simulink model "tetherDragForce_th"  (R2018b)
settings: Solver=VariableStepAuto  StartTime=0.0  StopTime=0  RelTol=1e-3
values from neighbouring files (symbols this model uses):
  flow = [1 0 0]'    [tetherDragForce_ts.m]
  R1_o = [0 0 0]'    [tetherDragForce_ts.m]
  Ri_o = zeros(3,N-2)    [tetherDragForce_ts.m]
  Rn_o = [0 0 100]'    [tetherDragForce_ts.m]
  V1_o = [0 0 0]'    [tetherDragForce_ts.m]
  Vi_o = zeros(size(Ri_o))    [tetherDragForce_ts.m]
  Vn_o = [0 0 0]'    [tetherDragForce_ts.m]
libraries: tetherDragForce_ul x1
settings Model: Creator=asiddiq2  LastModifiedBy=asiddiq2

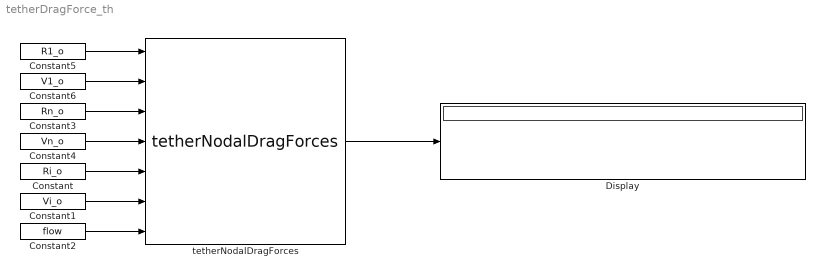
== system tetherDragForce_th ==
  Constant : Constant  Value=Ri_o  VectorParams1D=off
  Constant1 : Constant  Value=Vi_o  VectorParams1D=off
  Constant2 : Constant  Value=flow  VectorParams1D=off
  Constant3 : Constant  Value=Rn_o  VectorParams1D=off
  Constant4 : Constant  Value=Vn_o  VectorParams1D=off
  Constant5 : Constant  Value=R1_o  VectorParams1D=off
  Constant6 : Constant  Value=V1_o  VectorParams1D=off
  Display : Display
  tetherNodalDragForces : tetherDragForce_ul/tetherNodalDragForces  rhoFluid=rho_fluid  numNode=N  diaTether=dia_t  CdTether=Cd
  wires:
  Constant2/1 -> tetherNodalDragForces/7
  tetherNodalDragForces/1 -> Display/1
  Constant3/1 -> tetherNodalDragForces/3
  Constant5/1 -> tetherNodalDragForces/1
  Constant6/1 -> tetherNodalDragForces/2
  Constant4/1 -> tetherNodalDragForces/4
  Constant/1 -> tetherNodalDragForces/5
  Constant1/1 -> tetherNodalDragForces/6
